simulink library "BLDC_controller_Lib"  (R2017b)
settings: Solver=VariableStepAuto  StartTime=0.0  StopTime=10.0  RelTol=1e-3
libraries: BLDC_controller_Lib x9, simulink x9
settings Model: Creator=37ef  LastModifiedBy=eferu

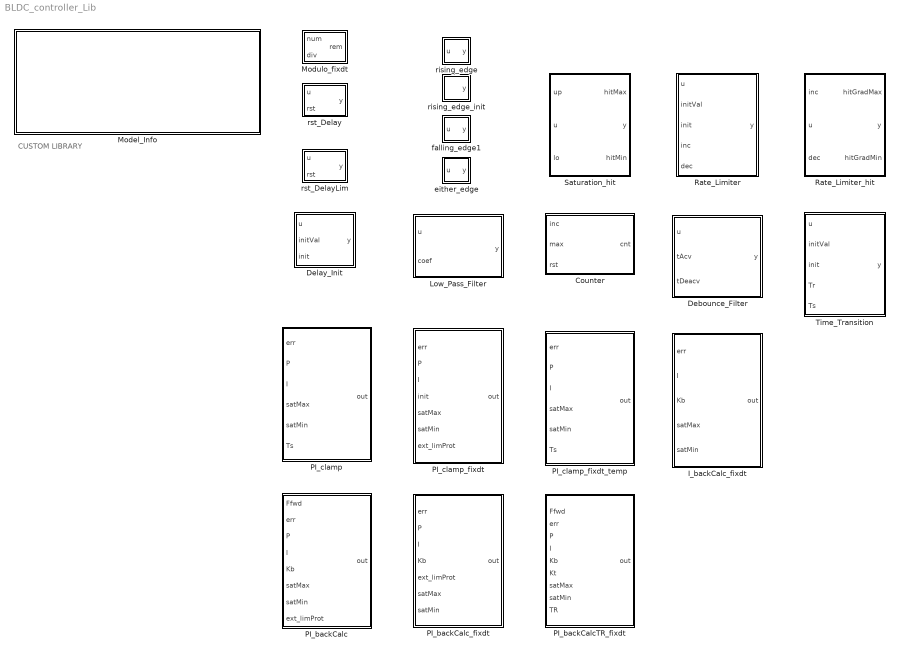
== system BLDC_controller_Lib ==
  note: CUSTOM LIBRARY
  Counter : Subsystem  TreatAsAtomicUnit=on  mask{z_cntInit=0}
      mask prompts: z_cntInit "Insert initial counter value"
      settings: AttributesFormatString=Ini=%<z_cntInit>  RTWFcnNameOpts=Use subsystem name
      mask Display: plot(0.15+[0.1,0.1],[0.1,0.9],[0.08,0.1,0.12]+0.15,[0.88,0.9,0.88],[0.25,0.8],[0.1,0.1],[0.88,0.9,0.88]-0.1,[0.08,0.1,0.12],0.05+[0.2,0.3,0.3,0.4,0.4,0.5,0.5,0.6,0.6,0.7],1.5*([0.1,0.1,0.2,0.2,0.3,0.3,0.4,0.4,0.5,0.5]-0.1)+0.1)
  Debounce_Filter : Subsystem  TreatAsAtomicUnit=on
      mask help:
      | This block implements a debounce filter.
      | The input and the output are boolean.
      | • Output will be 1 if input equals 1 during at least tAcv
      | • Output will be 0 if input equals 0 during at least tDeacv
      | ► Note that tAcv and tDeacv are integer numbers, represeting the number of time samples for Activation and Deactivation, respectively.
      settings: RTWFcnNameOpts=Use subsystem name
      mask Display:
      | plot([0.10 0.20 0.20 0.22 0.22 0.24 0.24 0.26 0.26 0.28 0.28 0.7 0.7 0.72 0.72 0.74 0.74 0.76 0.76 0.78 0.78 0.9],0.2+0.75*[0.55 0.55 0.9 0.9 0.55 0.55 0.9 0.9 0.55 0.55 0.9 0.9 0.55 0.55 0.9 0.9 0.55 0.55 0.9 0.9 0.55 0.55])
      | 
      | plot([0.10 0.28 0.28 0.78 0.78 0.90],0.2+0.7*[0.1 0.1 0.45 0.45 0.1 0.1])
  Delay_Init : Subsystem  mask{initVal=0}
      mask prompts: initVal "Initial value at program start"
      settings: AttributesFormatString=Ini=%<initVal>
      mask Display: dpoly(1,[1 0],'z')
  I_backCalc_fixdt : Subsystem  TreatAsAtomicUnit=on  mask{yInit=0}
      mask prompts: yInit "Initial output"
      settings: AttributesFormatString=Ini=%<yInit>  RTWFcnNameOpts=Use subsystem name
      mask Display: disp('I(z)')
  Low_Pass_Filter : Subsystem  TreatAsAtomicUnit=on
      settings: RTWFcnNameOpts=Use subsystem name
      mask Display:
      | plot(0,0,100,100, ...
      | [73,75,73,75,25,25,28,25,22,25],[18,20,22,20,20,84,82,84,82,84], ...
      | [25,33,33,72],[20,20,70,70],[33,34,36,39,44,50,56,66,73],[20,25,33,43,55,63,66,70,70]);
      | text(50,40,'coef'),
  Model_Info : Subsystem
      mask DialogControl DescGroupVar Prompt: Model info
      mask DialogControl DescTextVar Prompt: This mask gives quick information about the model.
      mask Display:
      | info = Simulink.MDLInfo(bdroot);
      | file = dir([bdroot '.slx']);
      | % image('logo.png', [0.48, 0.55, 0.5, 0.4]);
      | text(0.05, 0.5, [...
      |         'MODEL INFO \n\n' ...
      |         'Version: ' info.ModelVersion '\n' ...
      |         'Author: ' 'Emanuel Feru' '\n' ...
      |         'Last modified by: ' info.LastModifiedBy '\n' ...
      |         'Last update: ' file.date '\n\n'], ...
      |         'horizontalAlignment', 'left', ...
      |         'verticalAlignment', 'middle');
      | 
      | color('blue');
      | text(0.95, 0.08, [...
      |         'Copyright © 2019-2021 Emanuel FERU'], ...
      |         'horizontalAlignment', 'right', ...
      |         'verticalAlignment', 'bottom');
  Modulo_fixdt : Subsystem
  PI_backCalc : Subsystem  TreatAsAtomicUnit=on
      settings: RTWFcnNameOpts=Use subsystem name
      mask Display: disp('PI(z)')
  PI_backCalcTR_fixdt : Subsystem  TreatAsAtomicUnit=on
      settings: RTWFcnNameOpts=Use subsystem name
      mask Display: disp('PI(z)')
  PI_backCalc_fixdt : Subsystem  TreatAsAtomicUnit=on
      settings: RTWFcnNameOpts=Use subsystem name
      mask Display: disp('PI(z)')
  PI_clamp : Subsystem  TreatAsAtomicUnit=on
      settings: RTWFcnNameOpts=Use subsystem name
      mask Display: disp('PI(z)')
  PI_clamp_fixdt : Subsystem  TreatAsAtomicUnit=on
      settings: RTWFcnNameOpts=Use subsystem name
      mask Display: disp('PI(z)')
  PI_clamp_fixdt_temp : Subsystem  TreatAsAtomicUnit=on
      settings: RTWFcnNameOpts=Use subsystem name
      mask Display: disp('PI(z)')
  Rate_Limiter : Subsystem  TreatAsAtomicUnit=on
      settings: RTWFcnNameOpts=Use subsystem name
      mask Display: plot([0.15 0.85],[0.5 0.5],[0.5 0.5],[0.1 0.9],[0.25 0.75],[0.1 0.9])
  Rate_Limiter_hit : Subsystem  TreatAsAtomicUnit=on
      settings: RTWFcnNameOpts=Use subsystem name
      mask Display: plot([0.15 0.85],[0.5 0.5],[0.5 0.5],[0.1 0.9],[0.25 0.75],[0.1 0.9])
  Saturation_hit : Subsystem
      mask Display: plot([0.2 0.8],[0.5 0.5],[0.5 0.5],[0.05 0.95],[0.2 0.3 0.7 0.8],[0.05 0.05 0.95 0.95])
  Time_Transition : Subsystem  TreatAsAtomicUnit=on  mask{eps=5}
      mask prompts: eps "Convergence tolerance (eps)"
      mask help:
      | This block can be used to avoid discontinuity between a new input (discontinuous) and the previous output.
      |
      | When the input "init" is triggered, the error between "u" and "initVal" is set. This error is then reduced to 0 with respect to the transition time "Tr". When the error goes below a certain tolerance "eps", then the transition is finished.
      |
      | Once the error has been completely canceled (reduced to 0), then the output is equal to the input (without any slope constraint).
      settings: AttributesFormatString=eps=%<eps>  RTWFcnNameOpts=Use subsystem name
      mask Display:
      | plot(0,0,100,100,[88,90,88,90,29,29,31,29,27,29],[19,20,21,20,20,84,82,84,82,84]-5,...
      |     [35,40,50,60,70,85],[50,51,54,60,70,85]-5,[35,40,50,60,70,85],[30,35,45,56,70,85]-5);
      | text(35,22,'← Tr →');
  either_edge : Subsystem  StopFcn=%tagged  TreatAsAtomicUnit=on  mask(Either edge detection){}
      mask help:
      | Rising or falling edge detection for a logic signal.
      | When a rising or a falling edge on the input signal is detected, the output switches to 1 during one time step.
      mask Display: plot(0,0,100,100, [50 75 75 90], [90 90 10 10], [65 75 85], [55 45 55], [10 25 25 50], [10 10 90 90], [15 25 35], [45 55 45] )
  falling_edge1 : Subsystem  StopFcn=%tagged  TreatAsAtomicUnit=on  mask(Falling edge detection){}
      mask help:
      | Falling edge detection for a logic signal.
      | When a falling edge on the input signal is detected, the output switches to 1 during one time step.
      mask Display: plot(0,0,100,100, [20 50 50 80], [90 90 10 10], [40 50 60], [55 45 55] )
  rising_edge : Subsystem  StopFcn=%tagged  TreatAsAtomicUnit=on  mask(Rising edge detection){}
      mask help:
      | Rising edge detection for a logic signal.
      | When a rising edge on the input signal is detected, the output switches to 1 during one time step.
      mask Display: plot(0,0,100,100, [20 50 50 80], [10 10 90 90], [40 50 60], [45 55 45] )
  rising_edge_init : Subsystem  StopFcn=%tagged  TreatAsAtomicUnit=on  mask(Rising edge init){}
      mask help:
      | Rising edge at init of the subsystem.
      | This block can be used for example in action subsystem to create a trig when function is called.
      mask Display: plot(0,0,100,100, [20 50 50 80], [10 10 90 90], [40 50 60], [45 55 45] )
  rst_Delay : Subsystem  mask{initVal=0}
      mask prompts: initVal "Initial value at program start"
      settings: AttributesFormatString=Ini=%<InitVal>
      mask Display: dpoly(1,[1 0],'z')
  rst_DelayLim : Subsystem  mask{z_cntMaxLim=200}
      mask prompts: z_cntMaxLim "Maximum counter limit"
      settings: AttributesFormatString=Ini=%<z_cntMaxLim>
      mask Display: dpoly(1,[1 0],'z')

== system BLDC_controller_Lib/Counter ==
  inc : Inport
  max : Inport  Port=2
  rst : Inport  Port=3
  MinMax : MinMax  Inputs=2
  Sum1 : Sum  Inputs=|++  RndMeth=Simplest  InputSameDT=on  OutDataTypeStr=Inherit: Same as first input
  rst_Delay : BLDC_controller_Lib/rst_Delay  initVal=z_cntInit
      settings: AttributesFormatString=Ini=%<InitVal>
  cnt : Outport
  wires:
  inc/1 -> Sum1/1
  rst/1 -> rst_Delay/2
  Sum1/1 -> cnt/1, MinMax/1
  max/1 -> MinMax/2
  MinMax/1 -> rst_Delay/1
  rst_Delay/1 -> Sum1/2

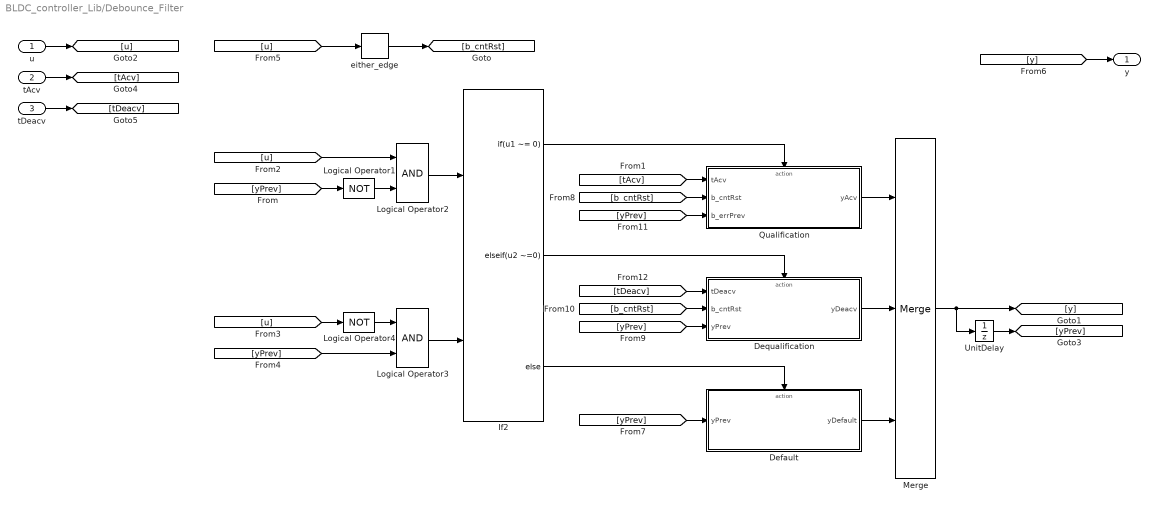
== system BLDC_controller_Lib/Debounce_Filter ==
  u : Inport
  tAcv : Inport  Port=2
  tDeacv : Inport  Port=3
  Default : Subsystem
  Dequalification : Subsystem
  If2 : If  NumInputs=2  IfExpression=u1 ~= 0  ElseIfExpressions=u2 ~=0
  Logical Operator1 : Logic  Operator=NOT  AllPortsSameDT=off  OutDataTypeStr=boolean
  Logical Operator2 : Logic  AllPortsSameDT=off  OutDataTypeStr=boolean
  Logical Operator3 : Logic  AllPortsSameDT=off  OutDataTypeStr=boolean
  Logical Operator4 : Logic  Operator=NOT  AllPortsSameDT=off  OutDataTypeStr=boolean
  Merge : Merge  Inputs=3
  Qualification : Subsystem
  UnitDelay : UnitDelay  SampleTime=-1
      settings: AttributesFormatString=Ini=%<X0>
  either_edge : BLDC_controller_Lib/either_edge
  y : Outport
  wires:
  Logical Operator2/1 -> If2/1
  Logical Operator3/1 -> If2/2
  [b_cntRst] -> Dequalification/2(b_cntRst)
  [yPrev] -> Logical Operator3/2
  Logical Operator4/1 -> Logical Operator3/1
  [tDeacv] -> Dequalification/1(tDeacv)
  Merge/1 -> UnitDelay/1, [y]
  UnitDelay/1 -> [yPrev]
  [b_cntRst] -> Qualification/2(b_cntRst)
  [tAcv] -> Qualification/1(tAcv)
  Dequalification/1(yDeacv) -> Merge/2
  Default/1(yDefault) -> Merge/3
  [yPrev] -> Qualification/3(b_errPrev)
  If2/2 -> Dequalification/Action
  [yPrev] -> Default/1(yPrev)
  [u] -> either_edge/1
  [y] -> y/1
  u/1 -> [u]
  If2/3 -> Default/Action
  [yPrev] -> Dequalification/3(yPrev)
  [u] -> Logical Operator4/1
  [yPrev] -> Logical Operator1/1
  Logical Operator1/1 -> Logical Operator2/2
  [u] -> Logical Operator2/1
  Qualification/1(yAcv) -> Merge/1
  If2/1 -> Qualification/Action
  tAcv/1 -> [tAcv]
  tDeacv/1 -> [tDeacv]
  either_edge/1 -> [b_cntRst]

== system BLDC_controller_Lib/Delay_Init ==
  u : Inport
  initVal : Inport  Port=2
  init : Inport  Port=3
  Switch1 : Switch  Criteria=u2 ~= 0  OutDataTypeStr=Inherit: Inherit via back propagation  RndMeth=Simplest  InputSameDT=on
  Switch2 : Switch  Criteria=u2 ~= 0  OutDataTypeStr=Inherit: Inherit via back propagation  RndMeth=Simplest  InputSameDT=on
  UnitDelay : UnitDelay  InitialCondition=initVal  SampleTime=-1
      settings: AttributesFormatString=Ini=%<X0>
  y : Outport
  wires:
  UnitDelay/1 -> Switch1/3
  Switch1/1 -> y/1
  init/1 -> Switch1/2, Switch2/2
  Switch2/1 -> UnitDelay/1
  u/1 -> Switch2/3
  initVal/1 -> Switch2/1, Switch1/1

== system BLDC_controller_Lib/I_backCalc_fixdt ==
  err : Inport
  I : Inport  Port=2
  Kb : Inport  Port=3
  satMax : Inport  Port=4
  satMin : Inport  Port=5
  Divide1 : Product  Inputs=**  RndMeth=Simplest
  Divide2 : Product  Inputs=**  RndMeth=Simplest
  Integrator : Subsystem
  Saturation Dynamic1 : simulink/Discontinuities/Saturation Dynamic  OutMin=[]  OutMax=[]  OutDataTypeStr=Inherit: Same as second input  OutDataType=fixdt(1, 16)  OutScaling=2^-10  DoSatur=off
  Sum2 : Sum  RndMeth=Simplest  SaturateOnIntegerOverflow=on
  Sum3 : Sum  Inputs=-+|  RndMeth=Simplest
  UnitDelay : UnitDelay  SampleTime=-1
      settings: AttributesFormatString=Ini=%<X0>
  out : Outport
  wires:
  satMin/1 -> Saturation Dynamic1/3
  satMax/1 -> Saturation Dynamic1/1
  I/1 -> Divide2/2
  err/1 -> Divide2/1
  Saturation Dynamic1/1 -> Sum3/2, out/1
  Integrator/1(y) -> Sum3/1, Saturation Dynamic1/2
  UnitDelay/1 -> Sum2/2
  Divide1/1 -> UnitDelay/1
  Sum3/1 -> Divide1/1
  Kb/1 -> Divide1/2
  Divide2/1 -> Sum2/1
  Sum2/1 -> Integrator/1(u)

== system BLDC_controller_Lib/Low_Pass_Filter ==
  u : Inport
  coef : Inport  Port=2
  Data Type Conversion : DataTypeConversion  OutDataTypeStr=fixdt(1,16,4)
  Divide3 : Product  Inputs=**  RndMeth=Simplest
  Sum2 : Sum  Inputs=+-  RndMeth=Simplest  SaturateOnIntegerOverflow=on  OutDataTypeStr=Inherit: Same as first input
  Sum3 : Sum  RndMeth=Simplest  OutDataTypeStr=Inherit: Same as first input
  UnitDelay1 : UnitDelay  SampleTime=-1
  y : Outport
  wires:
  Sum3/1 -> Data Type Conversion/1, UnitDelay1/1
  Sum2/1 -> Divide3/2
  UnitDelay1/1 -> Sum3/2, Sum2/2
  Data Type Conversion/1 -> y/1
  u/1 -> Sum2/1
  Divide3/1 -> Sum3/1
  coef/1 -> Divide3/1

== system BLDC_controller_Lib/Model_Info ==

== system BLDC_controller_Lib/Modulo_fixdt ==
  note: Modulo implementation: rem = num - div*(num/div)
      | Note : Division and multiplier has the setting 'Floor'
  num : Inport
  div : Inport  Port=2
  Divide2 : Product  Inputs=*/  OutDataTypeStr=fixdt(1,16,0)
  Divide3 : Product  Inputs=**  OutDataTypeStr=Inherit: Same as first input
  Sum3 : Sum  Inputs=|+-  RndMeth=Simplest  OutDataTypeStr=Inherit: Same as first input
  rem : Outport
  wires:
  Divide3/1 -> Sum3/2
  num/1 -> Divide2/1, Sum3/1
  Sum3/1 -> rem/1
  div/1 -> Divide2/2, Divide3/2
  Divide2/1 -> Divide3/1

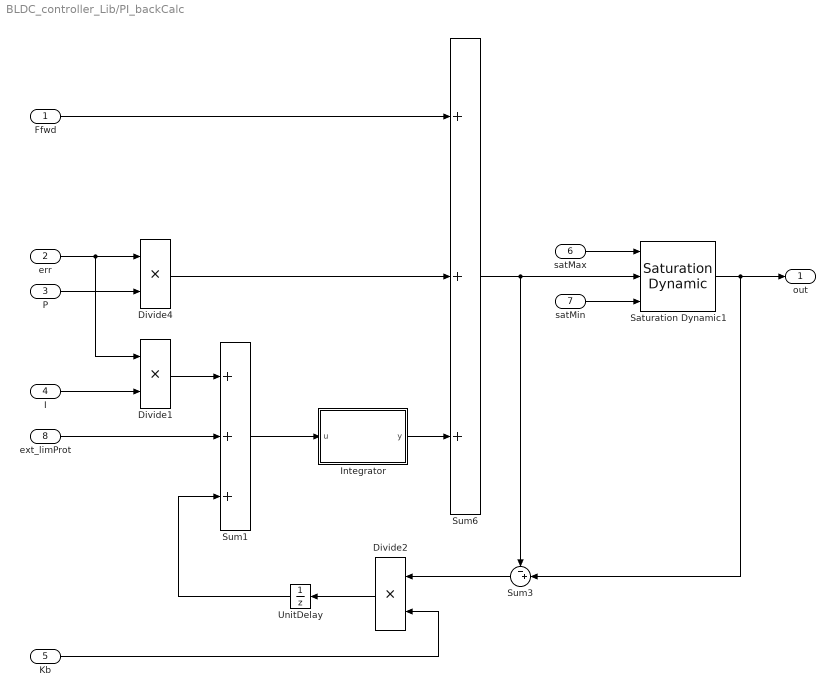
== system BLDC_controller_Lib/PI_backCalc ==
  Ffwd : Inport
  err : Inport  Port=2
  P : Inport  Port=3
  I : Inport  Port=4
  Kb : Inport  Port=5
  satMax : Inport  Port=6
  satMin : Inport  Port=7
  ext_limProt : Inport  Port=8
  Divide1 : Product  Inputs=**  RndMeth=Simplest
  Divide2 : Product  Inputs=**  RndMeth=Simplest
  Divide4 : Product  Inputs=**  RndMeth=Simplest
  Integrator : Subsystem
  Saturation Dynamic1 : simulink/Discontinuities/Saturation Dynamic  OutMin=[]  OutMax=[]  OutDataTypeStr=Inherit: Same as second input  OutDataType=fixdt(1, 16)  OutScaling=2^-10  DoSatur=off
  Sum1 : Sum  Inputs=+++  OutDataTypeStr=Inherit: Inherit via back propagation  RndMeth=Simplest  SaturateOnIntegerOverflow=on
  Sum3 : Sum  Inputs=-+|  OutDataTypeStr=Inherit: Inherit via back propagation  RndMeth=Simplest  SaturateOnIntegerOverflow=on
  Sum6 : Sum  Inputs=+++  OutDataTypeStr=single  RndMeth=Simplest  SaturateOnIntegerOverflow=on
  UnitDelay : UnitDelay  SampleTime=-1
      settings: AttributesFormatString=Ini=%<X0>
  out : Outport
  wires:
  I/1 -> Divide1/2
  P/1 -> Divide4/2
  Integrator/1(y) -> Sum6/3
  Saturation Dynamic1/1 -> Sum3/2, out/1
  Sum1/1 -> Integrator/1(u)
  Divide4/1 -> Sum6/2
  err/1 -> Divide1/1, Divide4/1
  satMax/1 -> Saturation Dynamic1/1
  Sum6/1 -> Sum3/1, Saturation Dynamic1/2
  satMin/1 -> Saturation Dynamic1/3
  Divide1/1 -> Sum1/1
  UnitDelay/1 -> Sum1/3
  Divide2/1 -> UnitDelay/1
  Sum3/1 -> Divide2/1
  Kb/1 -> Divide2/2
  ext_limProt/1 -> Sum1/2
  Ffwd/1 -> Sum6/1

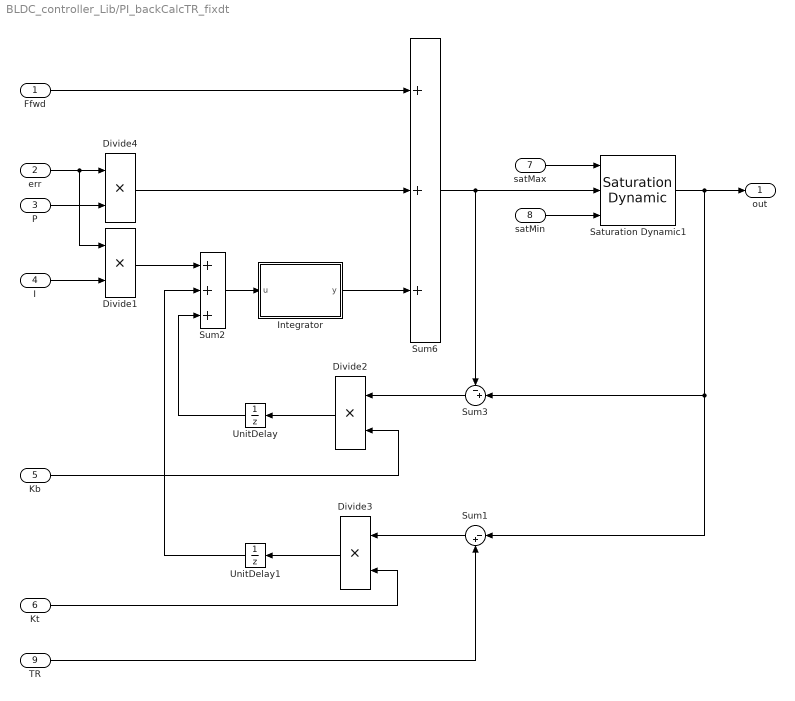
== system BLDC_controller_Lib/PI_backCalcTR_fixdt ==
  Ffwd : Inport
  err : Inport  Port=2
  P : Inport  Port=3
  I : Inport  Port=4
  Kb : Inport  Port=5
  Kt : Inport  Port=6
  satMax : Inport  Port=7
  satMin : Inport  Port=8
  TR : Inport  Port=9
  Divide{1..4} (4 alike) : Product  Inputs=**  RndMeth=Simplest
  Integrator : Subsystem
  Saturation Dynamic1 : simulink/Discontinuities/Saturation Dynamic  OutMin=[]  OutMax=[]  OutDataTypeStr=Inherit: Same as second input  OutDataType=fixdt(1, 16)  OutScaling=2^-10  DoSatur=off
  Sum1 : Sum  Inputs=|-+  RndMeth=Simplest  SaturateOnIntegerOverflow=on
  Sum2 : Sum  Inputs=+++  RndMeth=Simplest  SaturateOnIntegerOverflow=on
  Sum3 : Sum  Inputs=-+|  RndMeth=Simplest  SaturateOnIntegerOverflow=on
  Sum6 : Sum  Inputs=+++  OutDataTypeStr=fixdt(1,16,4)  RndMeth=Simplest  SaturateOnIntegerOverflow=on
  UnitDelay : UnitDelay  SampleTime=-1
      settings: AttributesFormatString=Ini=%<X0>
  UnitDelay1 : UnitDelay  SampleTime=-1
      settings: AttributesFormatString=Ini=%<X0>
  out : Outport
  wires:
  Sum2/1 -> Integrator/1(u)
  Kb/1 -> Divide2/2
  Saturation Dynamic1/1 -> out/1, Sum3/2, Sum1/1
  Sum6/1 -> Sum3/1, Saturation Dynamic1/2
  UnitDelay/1 -> Sum2/3
  Sum3/1 -> Divide2/1
  Divide2/1 -> UnitDelay/1
  Divide1/1 -> Sum2/1
  I/1 -> Divide1/2
  err/1 -> Divide1/1, Divide4/1
  Integrator/1(y) -> Sum6/3
  satMax/1 -> Saturation Dynamic1/1
  Divide4/1 -> Sum6/2
  satMin/1 -> Saturation Dynamic1/3
  P/1 -> Divide4/2
  Kt/1 -> Divide3/2
  Divide3/1 -> UnitDelay1/1
  Sum1/1 -> Divide3/1
  TR/1 -> Sum1/2
  UnitDelay1/1 -> Sum2/2
  Ffwd/1 -> Sum6/1

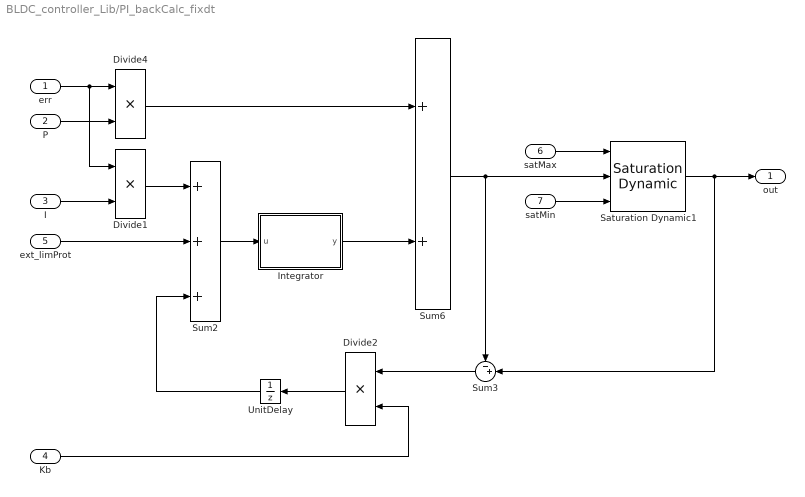
== system BLDC_controller_Lib/PI_backCalc_fixdt ==
  err : Inport
  P : Inport  Port=2
  I : Inport  Port=3
  Kb : Inport  Port=4
  ext_limProt : Inport  Port=5
  satMax : Inport  Port=6
  satMin : Inport  Port=7
  Divide1 : Product  Inputs=**  RndMeth=Simplest  SaturateOnIntegerOverflow=on
  Divide2 : Product  Inputs=**  RndMeth=Simplest
  Divide4 : Product  Inputs=**  OutDataTypeStr=fixdt(1,16,5)  RndMeth=Simplest  SaturateOnIntegerOverflow=on
  Integrator : Subsystem
  Saturation Dynamic1 : simulink/Discontinuities/Saturation Dynamic  OutMin=[]  OutMax=[]  OutDataTypeStr=Inherit: Same as second input  OutDataType=fixdt(1, 16)  OutScaling=2^-10  DoSatur=off
  Sum2 : Sum  Inputs=+++  RndMeth=Simplest  SaturateOnIntegerOverflow=on
  Sum3 : Sum  Inputs=-+|  RndMeth=Simplest
  Sum6 : Sum  OutDataTypeStr=fixdt(1,16,4)  RndMeth=Simplest  SaturateOnIntegerOverflow=on
  UnitDelay : UnitDelay  SampleTime=-1
      settings: AttributesFormatString=Ini=%<X0>
  out : Outport
  wires:
  ext_limProt/1 -> Sum2/2
  P/1 -> Divide4/2
  satMin/1 -> Saturation Dynamic1/3
  satMax/1 -> Saturation Dynamic1/1
  err/1 -> Divide4/1, Divide1/1
  I/1 -> Divide1/2
  Divide1/1 -> Sum2/1
  Divide2/1 -> UnitDelay/1
  Sum3/1 -> Divide2/1
  UnitDelay/1 -> Sum2/3
  Sum6/1 -> Saturation Dynamic1/2, Sum3/1
  Saturation Dynamic1/1 -> Sum3/2, out/1
  Kb/1 -> Divide2/2
  Sum2/1 -> Integrator/1(u)
  Integrator/1(y) -> Sum6/2
  Divide4/1 -> Sum6/1

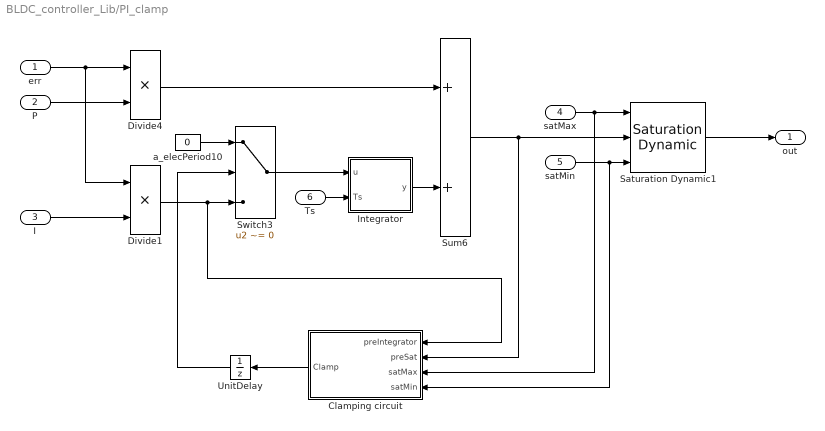
== system BLDC_controller_Lib/PI_clamp ==
  err : Inport
  P : Inport  Port=2
  I : Inport  Port=3
  satMax : Inport  Port=4
  satMin : Inport  Port=5
  Ts : Inport  Port=6
  Clamping circuit : Subsystem
  Divide1 : Product  Inputs=**  RndMeth=Simplest
  Divide4 : Product  Inputs=**  RndMeth=Simplest
  Integrator : Subsystem
  Saturation Dynamic1 : simulink/Discontinuities/Saturation Dynamic  OutMin=[]  OutMax=[]  OutDataTypeStr=Inherit: Same as second input  OutDataType=fixdt(1, 16)  OutScaling=2^-10  DoSatur=off
  Sum6 : Sum  OutDataTypeStr=single  RndMeth=Simplest  SaturateOnIntegerOverflow=on
  Switch3 : Switch  Criteria=u2 ~= 0  OutDataTypeStr=Inherit: Inherit via back propagation  RndMeth=Zero
  UnitDelay : UnitDelay  SampleTime=-1
      settings: AttributesFormatString=Ini=%<X0>
  a_elecPeriod10 : Constant  Value=0  OutDataTypeStr=Inherit: Inherit via back propagation
  out : Outport
  wires:
  satMin/1 -> Saturation Dynamic1/3, Clamping circuit/4(satMin)
  Sum6/1 -> Saturation Dynamic1/2, Clamping circuit/2(preSat)
  satMax/1 -> Saturation Dynamic1/1, Clamping circuit/3(satMax)
  Divide1/1 -> Switch3/3, Clamping circuit/1(preIntegrator)
  UnitDelay/1 -> Switch3/2
  Clamping circuit/1(Clamp) -> UnitDelay/1
  err/1 -> Divide4/1, Divide1/1
  Divide4/1 -> Sum6/1
  a_elecPeriod10/1 -> Switch3/1
  Switch3/1 -> Integrator/1(u)
  Saturation Dynamic1/1 -> out/1
  Integrator/1(y) -> Sum6/2
  P/1 -> Divide4/2
  I/1 -> Divide1/2
  Ts/1 -> Integrator/2(Ts)

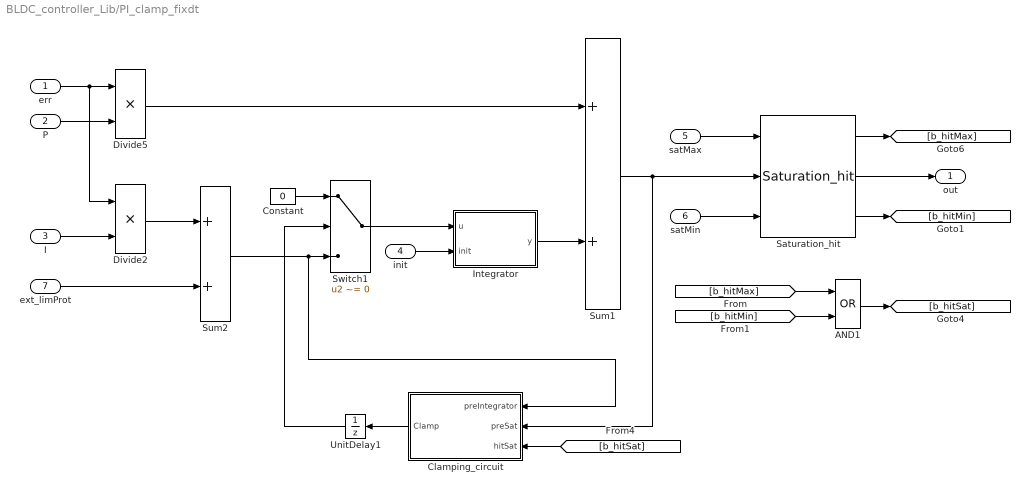
== system BLDC_controller_Lib/PI_clamp_fixdt ==
  err : Inport
  P : Inport  Port=2
  I : Inport  Port=3
  init : Inport  Port=4
  satMax : Inport  Port=5
  satMin : Inport  Port=6
  ext_limProt : Inport  Port=7
  AND1 : Logic  DisableCoverage=on  Operator=OR  OutDataTypeStr=boolean
  Clamping_circuit : Subsystem
  Constant : Constant  Value=0  OutDataTypeStr=Inherit: Inherit via back propagation
  Divide2 : Product  Inputs=**  RndMeth=Simplest
  Divide5 : Product  Inputs=**  OutDataTypeStr=fixdt(1,16,5)  RndMeth=Simplest  SaturateOnIntegerOverflow=on
  Integrator : Subsystem
  Saturation_hit : BLDC_controller_Lib/Saturation_hit  SystemSampleTime=-1
  Sum1 : Sum  OutDataTypeStr=fixdt(1,16,4)  RndMeth=Simplest  SaturateOnIntegerOverflow=on
  Sum2 : Sum  RndMeth=Simplest  SaturateOnIntegerOverflow=on
  Switch1 : Switch  Criteria=u2 ~= 0  OutDataTypeStr=Inherit: Inherit via back propagation  RndMeth=Zero
  UnitDelay1 : UnitDelay  SampleTime=-1
      settings: AttributesFormatString=Ini=%<X0>
  out : Outport
  wires:
  err/1 -> Divide5/1, Divide2/1
  ext_limProt/1 -> Sum2/2
  Divide2/1 -> Sum2/1
  Divide5/1 -> Sum1/1
  I/1 -> Divide2/2
  Integrator/1(y) -> Sum1/2
  P/1 -> Divide5/2
  satMax/1 -> Saturation_hit/1
  satMin/1 -> Saturation_hit/3
  Saturation_hit/1 -> [b_hitMax]
  Saturation_hit/3 -> [b_hitMin]
  Constant/1 -> Switch1/1
  Sum1/1 -> Clamping_circuit/2(preSat), Saturation_hit/2
  Sum2/1 -> Clamping_circuit/1(preIntegrator), Switch1/3
  Switch1/1 -> Integrator/1(u)
  Clamping_circuit/1(Clamp) -> UnitDelay1/1
  UnitDelay1/1 -> Switch1/2
  [b_hitMax] -> AND1/1
  [b_hitMin] -> AND1/2
  AND1/1 -> [b_hitSat]
  [b_hitSat] -> Clamping_circuit/3(hitSat)
  Saturation_hit/2 -> out/1
  init/1 -> Integrator/2(init)

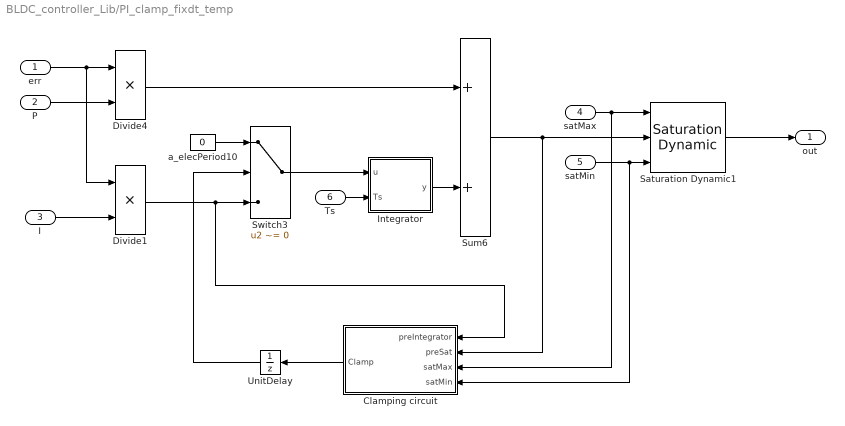
== system BLDC_controller_Lib/PI_clamp_fixdt_temp ==
  err : Inport
  P : Inport  Port=2
  I : Inport  Port=3
  satMax : Inport  Port=4
  satMin : Inport  Port=5
  Ts : Inport  Port=6
  Clamping circuit : Subsystem
  Divide1 : Product  Inputs=**  RndMeth=Simplest
  Divide4 : Product  Inputs=**  RndMeth=Simplest
  Integrator : Subsystem
  Saturation Dynamic1 : simulink/Discontinuities/Saturation Dynamic  OutMin=[]  OutMax=[]  OutDataTypeStr=Inherit: Same as second input  OutDataType=fixdt(1, 16)  OutScaling=2^-10  DoSatur=off
  Sum6 : Sum  OutDataTypeStr=fixdt(1,16,4)  RndMeth=Simplest  SaturateOnIntegerOverflow=on
  Switch3 : Switch  Criteria=u2 ~= 0  OutDataTypeStr=Inherit: Inherit via back propagation  RndMeth=Zero
  UnitDelay : UnitDelay  SampleTime=-1
      settings: AttributesFormatString=Ini=%<X0>
  a_elecPeriod10 : Constant  Value=0  OutDataTypeStr=Inherit: Inherit via back propagation
  out : Outport
  wires:
  UnitDelay/1 -> Switch3/2
  Clamping circuit/1(Clamp) -> UnitDelay/1
  Divide1/1 -> Switch3/3, Clamping circuit/1(preIntegrator)
  Switch3/1 -> Integrator/1(u)
  I/1 -> Divide1/2
  err/1 -> Divide4/1, Divide1/1
  Integrator/1(y) -> Sum6/2
  Sum6/1 -> Clamping circuit/2(preSat), Saturation Dynamic1/2
  satMax/1 -> Saturation Dynamic1/1, Clamping circuit/3(satMax)
  Divide4/1 -> Sum6/1
  satMin/1 -> Saturation Dynamic1/3, Clamping circuit/4(satMin)
  a_elecPeriod10/1 -> Switch3/1
  Saturation Dynamic1/1 -> out/1
  P/1 -> Divide4/2
  Ts/1 -> Integrator/2(Ts)

== system BLDC_controller_Lib/Rate_Limiter ==
  note: Rate Limiter
      | Note: The sample time must be included in the Increment and Decrement values.
  u : Inport
  initVal : Inport  Port=2
  init : Inport  Port=3
  inc : Inport  Port=4
  dec : Inport  Port=5
  Delay_Init1 : BLDC_controller_Lib/Delay_Init  initVal=0
  Saturation Dynamic : simulink/Discontinuities/Saturation Dynamic  OutMin=[]  OutMax=[]  OutDataTypeStr=Inherit: Same as second input  OutDataType=fixdt(1, 16)  OutScaling=2^-10  DoSatur=off
  Sum1 : Sum  Inputs=+-  RndMeth=Zero  OutDataTypeStr=Inherit: Same as first input
  Sum2 : Sum  RndMeth=Zero  OutDataTypeStr=Inherit: Same as first input
  y : Outport
  wires:
  Saturation Dynamic/1 -> Sum2/1
  initVal/1 -> Delay_Init1/2
  dec/1 -> Saturation Dynamic/3
  Sum1/1 -> Saturation Dynamic/2
  Sum2/1 -> y/1, Delay_Init1/1
  inc/1 -> Saturation Dynamic/1
  u/1 -> Sum1/1
  Delay_Init1/1 -> Sum2/2, Sum1/2
  init/1 -> Delay_Init1/3

== system BLDC_controller_Lib/Rate_Limiter_hit ==
  note: Rate Limiter
      | Note: The sample time must be included in the Increment and Decrement values.
  inc : Inport
  u : Inport  Port=2
  dec : Inport  Port=3
  Saturation_hit : BLDC_controller_Lib/Saturation_hit  SystemSampleTime=-1
  Sum1 : Sum  Inputs=+-  RndMeth=Zero  OutDataTypeStr=Inherit: Same as first input
  Sum2 : Sum  RndMeth=Zero  OutDataTypeStr=Inherit: Same as first input
  UnitDelay : UnitDelay  SampleTime=-1
      settings: AttributesFormatString=Ini=%<X0>
  hitGradMax : Outport
  y : Outport  Port=2
  hitGradMin : Outport  Port=3
  wires:
  UnitDelay/1 -> Sum1/2, Sum2/2
  u/1 -> Sum1/1
  inc/1 -> Saturation_hit/1
  Sum2/1 -> UnitDelay/1, y/1
  Sum1/1 -> Saturation_hit/2
  dec/1 -> Saturation_hit/3
  Saturation_hit/2 -> Sum2/1
  Saturation_hit/1 -> hitGradMax/1
  Saturation_hit/3 -> hitGradMin/1

== system BLDC_controller_Lib/Saturation_hit ==
  up : Inport
  u : Inport  Port=2
  lo : Inport  Port=3
  LowerRelop1 : RelationalOperator  DisableCoverage=on  Operator=>  OutDataTypeStr=boolean  RndMeth=Nearest
  Switch1 : Switch  Criteria=u2 ~= 0  OutDataTypeStr=Inherit: Inherit via back propagation  RndMeth=Zero
  Switch3 : Switch  Criteria=u2 ~= 0  OutDataTypeStr=Inherit: Inherit via back propagation  RndMeth=Zero
  UpperRelop : RelationalOperator  DisableCoverage=on  Operator=<  OutDataTypeStr=boolean  RndMeth=Nearest
  hitMax : Outport
  y : Outport  Port=2
  hitMin : Outport  Port=3
  wires:
  Switch1/1 -> y/1
  u/1 -> Switch3/3, LowerRelop1/1, UpperRelop/1
  up/1 -> LowerRelop1/2, Switch1/1
  UpperRelop/1 -> Switch3/2, hitMin/1
  LowerRelop1/1 -> hitMax/1, Switch1/2
  lo/1 -> Switch3/1, UpperRelop/2
  Switch3/1 -> Switch1/3

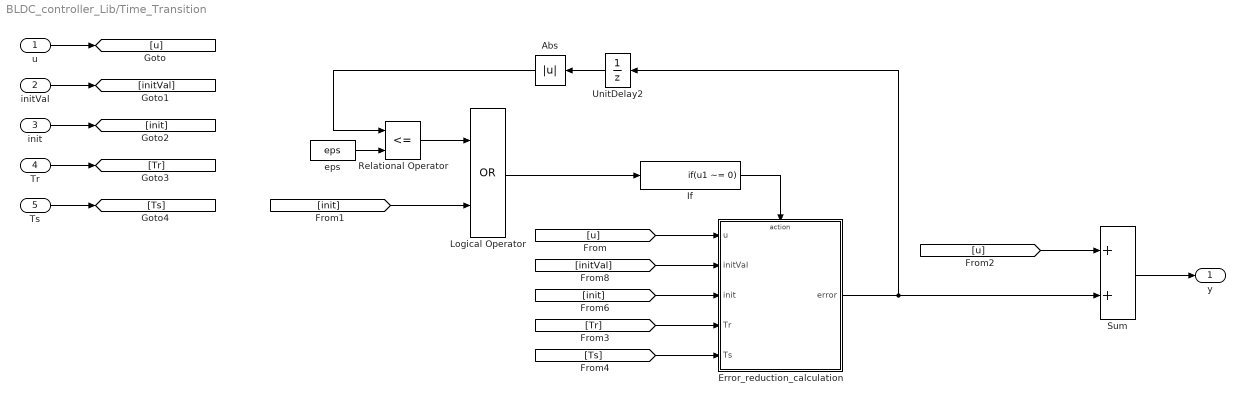
== system BLDC_controller_Lib/Time_Transition ==
  u : Inport
  initVal : Inport  Port=2
  init : Inport  Port=3
  Tr : Inport  Port=4
  Ts : Inport  Port=5
  Abs : Abs  RndMeth=Zero  SaturateOnIntegerOverflow=on
  Error_reduction_calculation : Subsystem  TreatAsAtomicUnit=on
  If : If  IfExpression=u1 ~= 0  ShowElse=off
  Logical Operator : Logic  Operator=OR  OutDataTypeStr=boolean
  Relational Operator : RelationalOperator  Operator=<=  OutDataTypeStr=boolean  RndMeth=Nearest  InputSameDT=on
  Sum : Sum  RndMeth=Zero  SaturateOnIntegerOverflow=on  OutDataTypeStr=Inherit: Same as first input
  UnitDelay2 : UnitDelay  SampleTime=-1
      settings: AttributesFormatString=Ini=%<X0>
  eps : Constant  Value=eps  OutDataTypeStr=Inherit: Inherit via back propagation
  y : Outport
  wires:
  eps/1 -> Relational Operator/2
  Error_reduction_calculation/1(error) -> Sum/2, UnitDelay2/1
  UnitDelay2/1 -> Abs/1
  Logical Operator/1 -> If/1
  [init] -> Logical Operator/2
  Relational Operator/1 -> Logical Operator/1
  If/1 -> Error_reduction_calculation/Action
  Abs/1 -> Relational Operator/1
  Sum/1 -> y/1
  u/1 -> [u]
  [u] -> Error_reduction_calculation/1(u)
  initVal/1 -> [initVal]
  [initVal] -> Error_reduction_calculation/2(initVal)
  [init] -> Error_reduction_calculation/3(init)
  init/1 -> [init]
  [Tr] -> Error_reduction_calculation/4(Tr)
  Tr/1 -> [Tr]
  Ts/1 -> [Ts]
  [Ts] -> Error_reduction_calculation/5(Ts)
  [u] -> Sum/1

== system BLDC_controller_Lib/either_edge ==
  u : Inport
  Relational Operator : RelationalOperator  Operator=~=  OutDataTypeStr=boolean  RndMeth=Nearest  InputSameDT=on
  UnitDelay : UnitDelay  SampleTime=-1
      settings: AttributesFormatString=Ini=%<X0>
  y : Outport
  wires:
  UnitDelay/1 -> Relational Operator/2
  Relational Operator/1 -> y/1
  u/1 -> UnitDelay/1, Relational Operator/1

== system BLDC_controller_Lib/falling_edge1 ==
  u : Inport
  Logical Operator : Logic  Tag=struct('inputs','2','comment',struct('text','','placement',1),'logdata',struct('maxnumvals',inf,'plotchannels',[],'loggingmode',3,'channels',1),'operator','AND','output',struct('variable','','description','','name','$S_$B','address','','class','default','type','Bool','unit',''),'scalingvalid',0,'date',733067.68453166669)  OutDataTypeStr=boolean
  Logical Operator1 : Logic  Tag=struct('inputs','1','comment',struct('text','','placement',1),'logdata',struct('maxnumvals',inf,'plotchannels',[],'loggingmode',3,'channels',1),'operator','NOT','output',struct('variable','','description','','name','$S_$B','address','','class','default','type','Bool','unit',''),'scalingvalid',0,'date',733067.68453201384)  Operator=NOT  Inputs=1  OutDataTypeStr=boolean
  UnitDelay : UnitDelay  SampleTime=-1
      settings: AttributesFormatString=Ini=%<X0>
  y : Outport
  wires:
  UnitDelay/1 -> Logical Operator/2
  Logical Operator1/1 -> Logical Operator/1
  u/1 -> UnitDelay/1, Logical Operator1/1
  Logical Operator/1 -> y/1

== system BLDC_controller_Lib/rising_edge ==
  u : Inport
  Logical Operator : Logic  Tag=struct('inputs','2','comment',struct('text','','placement',1),'logdata',struct('maxnumvals',inf,'plotchannels',[],'loggingmode',3,'channels',1),'operator','AND','output',struct('variable','','description','','name','$S_$B','address','','class','default','type','Bool','unit',''),'scalingvalid',0,'date',733067.68458487268)  OutDataTypeStr=boolean
  Logical Operator1 : Logic  Tag=struct('inputs','1','comment',struct('text','','placement',1),'logdata',struct('maxnumvals',inf,'plotchannels',[],'loggingmode',3,'channels',1),'operator','NOT','output',struct('variable','','description','','name','$S_$B','address','','class','default','type','Bool','unit',''),'scalingvalid',0,'date',733067.68458533566)  Operator=NOT  Inputs=1  OutDataTypeStr=boolean
  UnitDelay : UnitDelay  SampleTime=-1
      settings: AttributesFormatString=Ini=%<X0>
  y : Outport
  wires:
  UnitDelay/1 -> Logical Operator1/1
  Logical Operator1/1 -> Logical Operator/2
  u/1 -> Logical Operator/1, UnitDelay/1
  Logical Operator/1 -> y/1

== system BLDC_controller_Lib/rising_edge_init ==
  Constant : Constant  Value=0  OutDataTypeStr=boolean
  UnitDelay : UnitDelay  InitialCondition=1  SampleTime=-1
      settings: AttributesFormatString=Ini=%<X0>
  y : Outport
  wires:
  Constant/1 -> UnitDelay/1
  UnitDelay/1 -> y/1

== system BLDC_controller_Lib/rst_Delay ==
  u : Inport
  rst : Inport  Port=2
  Constant23 : Constant  Value=0  OutDataTypeStr=Inherit: Inherit via back propagation
  Switch1 : Switch  Criteria=u2 ~= 0  OutDataTypeStr=Inherit: Inherit via back propagation  RndMeth=Simplest
  UnitDelay : UnitDelay  InitialCondition=initVal  SampleTime=-1
      settings: AttributesFormatString=Ini=%<X0>
  y : Outport
  wires:
  Switch1/1 -> y/1
  u/1 -> UnitDelay/1
  UnitDelay/1 -> Switch1/3
  rst/1 -> Switch1/2
  Constant23/1 -> Switch1/1

== system BLDC_controller_Lib/rst_DelayLim ==
  u : Inport
  rst : Inport  Port=2
  Constant1 : Constant  Value=z_cntMaxLim  OutDataTypeStr=Inherit: Inherit via back propagation
  Constant23 : Constant  Value=0  OutDataTypeStr=Inherit: Inherit via back propagation
  Relational Operator1 : RelationalOperator  Operator=<  OutDataTypeStr=boolean  RndMeth=Simplest
  Switch1 : Switch  Criteria=u2 ~= 0  OutDataTypeStr=Inherit: Inherit via back propagation  RndMeth=Simplest
  Switch2 : Switch  Criteria=u2 ~= 0  OutDataTypeStr=Inherit: Inherit via back propagation  RndMeth=Simplest
  UnitDelay : UnitDelay  InitialCondition=z_cntMaxLim  SampleTime=-1
      settings: AttributesFormatString=Ini=%<X0>
  y : Outport
  wires:
  Switch1/1 -> y/1
  u/1 -> UnitDelay/1
  rst/1 -> Switch1/2
  Constant23/1 -> Switch1/1
  UnitDelay/1 -> Switch2/1, Relational Operator1/1
  Constant1/1 -> Switch2/3, Relational Operator1/2
  Relational Operator1/1 -> Switch2/2
  Switch2/1 -> Switch1/3

== system BLDC_controller_Lib/Debounce_Filter/Default ==
  note: Hold the previous value
  yPrev : Inport
  Action Port : ActionPort
  yDefault : Outport
  wires:
  yPrev/1 -> yDefault/1

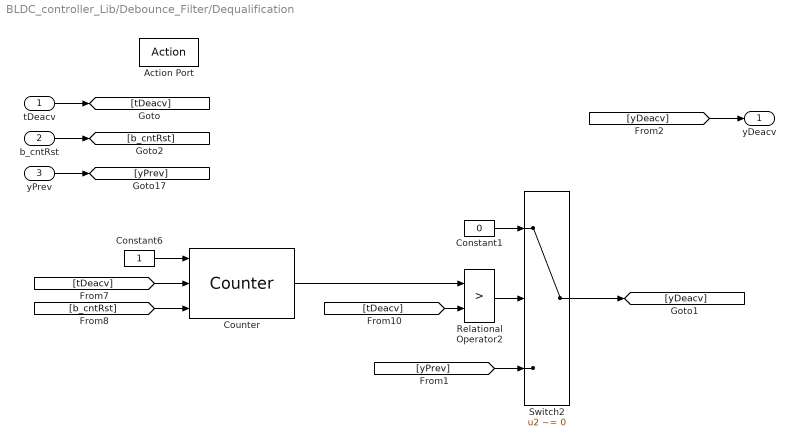
== system BLDC_controller_Lib/Debounce_Filter/Dequalification ==
  tDeacv : Inport
  b_cntRst : Inport  Port=2
  yPrev : Inport  Port=3
  Action Port : ActionPort
  Constant1 : Constant  Value=0  OutDataTypeStr=Inherit: Inherit via back propagation
  Constant6 : Constant  OutDataTypeStr=uint16
  Counter : BLDC_controller_Lib/Counter  z_cntInit=0
  Relational Operator2 : RelationalOperator  Operator=>  OutDataTypeStr=boolean  RndMeth=Simplest
  Switch2 : Switch  Criteria=u2 ~= 0  OutDataTypeStr=Inherit: Inherit via back propagation  RndMeth=Zero
  yDeacv : Outport
  wires:
  Counter/1 -> Relational Operator2/1
  Switch2/1 -> [yDeacv]
  [yPrev] -> Switch2/3
  Constant1/1 -> Switch2/1
  Relational Operator2/1 -> Switch2/2
  [tDeacv] -> Relational Operator2/2
  [b_cntRst] -> Counter/3
  [tDeacv] -> Counter/2
  Constant6/1 -> Counter/1
  yPrev/1 -> [yPrev]
  b_cntRst/1 -> [b_cntRst]
  tDeacv/1 -> [tDeacv]
  [yDeacv] -> yDeacv/1

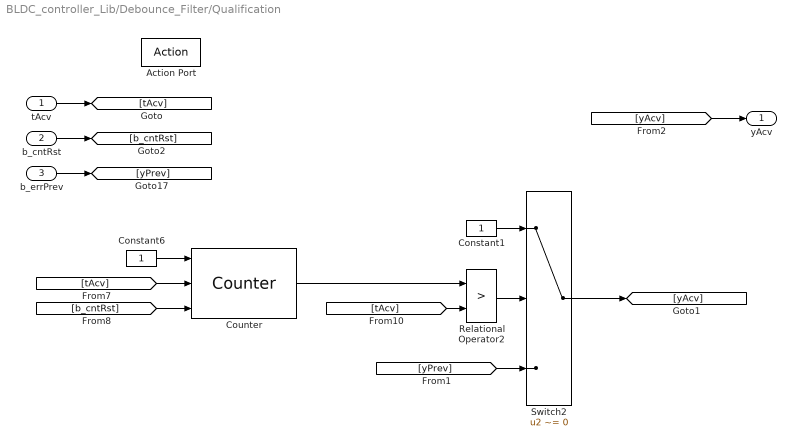
== system BLDC_controller_Lib/Debounce_Filter/Qualification ==
  tAcv : Inport
  b_cntRst : Inport  Port=2
  b_errPrev : Inport  Port=3
  Action Port : ActionPort
  Constant1 : Constant  OutDataTypeStr=Inherit: Inherit via back propagation
  Constant6 : Constant  OutDataTypeStr=uint16
  Counter : BLDC_controller_Lib/Counter  z_cntInit=0
  Relational Operator2 : RelationalOperator  Operator=>  OutDataTypeStr=boolean  RndMeth=Simplest
  Switch2 : Switch  Criteria=u2 ~= 0  OutDataTypeStr=Inherit: Inherit via back propagation  RndMeth=Zero
  yAcv : Outport
  wires:
  [yAcv] -> yAcv/1
  tAcv/1 -> [tAcv]
  b_cntRst/1 -> [b_cntRst]
  b_errPrev/1 -> [yPrev]
  Constant6/1 -> Counter/1
  [tAcv] -> Counter/2
  [b_cntRst] -> Counter/3
  [tAcv] -> Relational Operator2/2
  Relational Operator2/1 -> Switch2/2
  Constant1/1 -> Switch2/1
  [yPrev] -> Switch2/3
  Switch2/1 -> [yAcv]
  Counter/1 -> Relational Operator2/1

== system BLDC_controller_Lib/I_backCalc_fixdt/Integrator ==
  u : Inport
  Data Type Conversion1 : DataTypeConversion  OutDataTypeStr=fixdt(1,16,4)
  Sum1 : Sum  Inputs=|++  RndMeth=Simplest  OutDataTypeStr=Inherit: Same as first input
  UnitDelay : UnitDelay  InitialCondition=yInit  SampleTime=-1
      settings: AttributesFormatString=Ini=%<X0>
  y : Outport
  wires:
  Data Type Conversion1/1 -> y/1
  UnitDelay/1 -> Sum1/2
  Sum1/1 -> UnitDelay/1, Data Type Conversion1/1
  u/1 -> Sum1/1

== system BLDC_controller_Lib/PI_backCalc/Integrator ==
  u : Inport
  Sum1 : Sum  Inputs=|++  RndMeth=Simplest  OutDataTypeStr=Inherit: Same as first input
  UnitDelay : UnitDelay  SampleTime=-1
      settings: AttributesFormatString=Ini=%<X0>
  y : Outport
  wires:
  u/1 -> Sum1/1
  Sum1/1 -> UnitDelay/1, y/1
  UnitDelay/1 -> Sum1/2

== system BLDC_controller_Lib/PI_backCalcTR_fixdt/Integrator ==
  u : Inport
  Sum1 : Sum  Inputs=|++  RndMeth=Simplest  OutDataTypeStr=Inherit: Same as first input
  UnitDelay : UnitDelay  SampleTime=-1
      settings: AttributesFormatString=Ini=%<X0>
  y : Outport
  wires:
  UnitDelay/1 -> Sum1/2
  Sum1/1 -> UnitDelay/1, y/1
  u/1 -> Sum1/1

== system BLDC_controller_Lib/PI_backCalc_fixdt/Integrator ==
  u : Inport
  Data Type Conversion1 : DataTypeConversion  OutDataTypeStr=fixdt(1,16,4)
  Sum1 : Sum  Inputs=|++  RndMeth=Simplest  OutDataTypeStr=Inherit: Same as first input
  UnitDelay : UnitDelay  SampleTime=-1
      settings: AttributesFormatString=Ini=%<X0>
  y : Outport
  wires:
  u/1 -> Sum1/1
  Sum1/1 -> UnitDelay/1, Data Type Conversion1/1
  UnitDelay/1 -> Sum1/2
  Data Type Conversion1/1 -> y/1

== system BLDC_controller_Lib/PI_clamp/Clamping circuit ==
  preIntegrator : Inport  DisableCoverage=on
  preSat : Inport  DisableCoverage=on  Port=2
  satMax : Inport  DisableCoverage=on  Port=3
  satMin : Inport  DisableCoverage=on  Port=4
  AND : Logic  DisableCoverage=on
  DataTypeConv1 : DataTypeConversion  DisableCoverage=on  OutDataTypeStr=int8  RndMeth=Zero  LockScale=on
  DataTypeConv2 : DataTypeConversion  DisableCoverage=on  OutDataTypeStr=int8  RndMeth=Zero  LockScale=on
  Dead Zone Dynamic : simulink/Discontinuities/Dead Zone Dynamic
      settings: SourceProductName=Simulink  SourceProductBaseCode=SL
  Equal : RelationalOperator  DisableCoverage=on  Operator===  RndMeth=Zero  InputSameDT=on
  NotEqual : RelationalOperator  DisableCoverage=on  Operator=~=  RndMeth=Nearest  InputSameDT=on
  SignDeltaU : Signum  DisableCoverage=on
  SignDeltaU1 : Signum  DisableCoverage=on
  a_elecPeriod10 : Constant  Value=0  OutDataTypeStr=Inherit: Inherit via back propagation
  Clamp : Outport  DisableCoverage=on
  wires:
  preIntegrator/1 -> SignDeltaU1/1
  Dead Zone Dynamic/1 -> NotEqual/2, SignDeltaU/1
  SignDeltaU/1 -> DataTypeConv1/1
  DataTypeConv1/1 -> Equal/1
  SignDeltaU1/1 -> DataTypeConv2/1
  DataTypeConv2/1 -> Equal/2
  NotEqual/1 -> AND/1
  Equal/1 -> AND/2
  AND/1 -> Clamp/1
  a_elecPeriod10/1 -> NotEqual/1
  preSat/1 -> Dead Zone Dynamic/2
  satMax/1 -> Dead Zone Dynamic/1
  satMin/1 -> Dead Zone Dynamic/3

== system BLDC_controller_Lib/PI_clamp/Integrator ==
  u : Inport
  Ts : Inport  Port=2
  Divide2 : Product  Inputs=**  OutDataTypeStr=Inherit: Inherit via back propagation  RndMeth=Simplest
  Sum1 : Sum  Inputs=|++  RndMeth=Simplest  OutDataTypeStr=Inherit: Same as first input
  UnitDelay : UnitDelay  SampleTime=-1
      settings: AttributesFormatString=Ini=%<X0>
  y : Outport
  wires:
  UnitDelay/1 -> Sum1/2
  u/1 -> Divide2/1
  Sum1/1 -> UnitDelay/1, y/1
  Divide2/1 -> Sum1/1
  Ts/1 -> Divide2/2

== system BLDC_controller_Lib/PI_clamp_fixdt/Clamping_circuit ==
  preIntegrator : Inport  DisableCoverage=on
  preSat : Inport  DisableCoverage=on  Port=2
  hitSat : Inport  DisableCoverage=on  Port=3
  AND1 : Logic  DisableCoverage=on  OutDataTypeStr=boolean
  DataTypeConv3 : DataTypeConversion  DisableCoverage=on  OutDataTypeStr=int8  RndMeth=Zero  LockScale=on
  DataTypeConv4 : DataTypeConversion  DisableCoverage=on  OutDataTypeStr=int8  RndMeth=Zero  LockScale=on
  Equal1 : RelationalOperator  DisableCoverage=on  Operator===  RndMeth=Zero  InputSameDT=on
  SignDeltaU2 : Signum  DisableCoverage=on
  SignDeltaU3 : Signum  DisableCoverage=on
  Clamp : Outport  DisableCoverage=on
  wires:
  preIntegrator/1 -> SignDeltaU2/1
  preSat/1 -> SignDeltaU3/1
  SignDeltaU2/1 -> DataTypeConv3/1
  SignDeltaU3/1 -> DataTypeConv4/1
  DataTypeConv3/1 -> Equal1/1
  DataTypeConv4/1 -> Equal1/2
  Equal1/1 -> AND1/1
  AND1/1 -> Clamp/1
  hitSat/1 -> AND1/2

== system BLDC_controller_Lib/PI_clamp_fixdt/Integrator ==
  u : Inport
  init : Inport  Port=2
  Data Type Conversion1 : DataTypeConversion  OutDataTypeStr=fixdt(1,16,4)
  Resettable Delay : Delay  DelayLength=1  InitialConditionSource=Input port
      settings: InputPortMap=u0,p4
  Sum1 : Sum  Inputs=|++  RndMeth=Simplest  OutDataTypeStr=Inherit: Same as first input
  y : Outport
  wires:
  u/1 -> Sum1/1
  Sum1/1 -> Resettable Delay/1, Data Type Conversion1/1
  Resettable Delay/1 -> Sum1/2
  Data Type Conversion1/1 -> y/1
  init/1 -> Resettable Delay/2

== system BLDC_controller_Lib/PI_clamp_fixdt_temp/Clamping circuit ==
  preIntegrator : Inport  DisableCoverage=on
  preSat : Inport  DisableCoverage=on  Port=2
  satMax : Inport  DisableCoverage=on  Port=3
  satMin : Inport  DisableCoverage=on  Port=4
  AND : Logic  DisableCoverage=on
  DataTypeConv1 : DataTypeConversion  DisableCoverage=on  OutDataTypeStr=int8  RndMeth=Zero  LockScale=on
  DataTypeConv2 : DataTypeConversion  DisableCoverage=on  OutDataTypeStr=int8  RndMeth=Zero  LockScale=on
  Dead Zone Dynamic : simulink/Discontinuities/Dead Zone Dynamic
      settings: SourceProductName=Simulink  SourceProductBaseCode=SL
  Equal : RelationalOperator  DisableCoverage=on  Operator===  RndMeth=Zero  InputSameDT=on
  NotEqual : RelationalOperator  DisableCoverage=on  Operator=~=  RndMeth=Nearest  InputSameDT=on
  SignDeltaU : Signum  DisableCoverage=on
  SignDeltaU1 : Signum  DisableCoverage=on
  a_elecPeriod10 : Constant  Value=0  OutDataTypeStr=Inherit: Inherit via back propagation
  Clamp : Outport  DisableCoverage=on
  wires:
  satMin/1 -> Dead Zone Dynamic/3
  satMax/1 -> Dead Zone Dynamic/1
  preSat/1 -> Dead Zone Dynamic/2
  a_elecPeriod10/1 -> NotEqual/1
  AND/1 -> Clamp/1
  Equal/1 -> AND/2
  NotEqual/1 -> AND/1
  DataTypeConv2/1 -> Equal/2
  SignDeltaU1/1 -> DataTypeConv2/1
  DataTypeConv1/1 -> Equal/1
  SignDeltaU/1 -> DataTypeConv1/1
  Dead Zone Dynamic/1 -> SignDeltaU/1, NotEqual/2
  preIntegrator/1 -> SignDeltaU1/1

== system BLDC_controller_Lib/PI_clamp_fixdt_temp/Integrator ==
  u : Inport
  Ts : Inport  Port=2
  Divide2 : Product  Inputs=**  OutDataTypeStr=Inherit: Inherit via back propagation  RndMeth=Simplest
  Sum1 : Sum  Inputs=|++  RndMeth=Simplest  OutDataTypeStr=Inherit: Same as first input
  UnitDelay : UnitDelay  SampleTime=-1
      settings: AttributesFormatString=Ini=%<X0>
  y : Outport
  wires:
  UnitDelay/1 -> Sum1/2
  u/1 -> Divide2/1
  Sum1/1 -> UnitDelay/1, y/1
  Divide2/1 -> Sum1/1
  Ts/1 -> Divide2/2

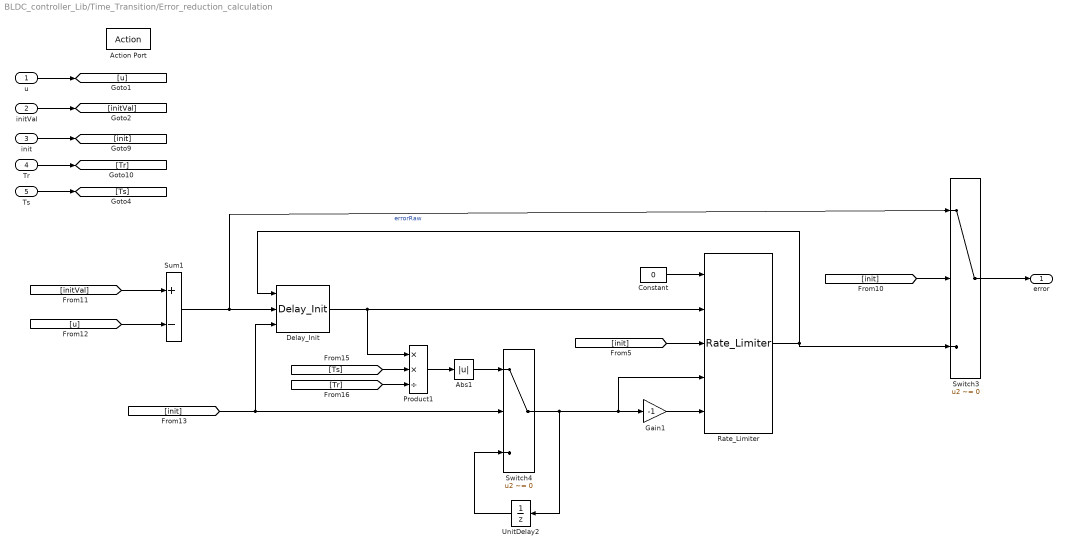
== system BLDC_controller_Lib/Time_Transition/Error_reduction_calculation ==
  u : Inport
  initVal : Inport  Port=2
  init : Inport  Port=3
  Tr : Inport  Port=4
  Ts : Inport  Port=5
  Action Port : ActionPort  InitializeStates=reset
  Abs1 : Abs  RndMeth=Zero  SaturateOnIntegerOverflow=on
  Constant : Constant  Value=0  OutDataTypeStr=Inherit: Inherit via back propagation
  Delay_Init : BLDC_controller_Lib/Delay_Init  initVal=0
      settings: AttributesFormatString=Ini=%<initVal>
  Gain1 : Gain  Gain=-1  RndMeth=Zero  OutDataTypeStr=Inherit: Same as input
  Product1 : Product  Tag=struct('comment',struct('text','','placement',1),'logdata',struct('maxnumvals',inf,'plotchannels',[],'loggingmode',3,'channels',1),'output',struct('variable','','description','','name','$S_$B','width',1,'address','','max',NaN,'min',NaN,'class','default','type','CONTINUOUS','scaling','','lsb',1,'offset',0,'arb',0,'freeze',1,'unit','','autoscalingmode',1,'lowerheadroom',1,'upperheadroom',1,'headroomunit','bit','keepdatatype',1,'checkmin',0,'checkmax',0,'castoutput',0,'show',0),'inputs','**','exceptionhandling',1,'scalingvalid',0,'date',730486)  Inputs=**/  SaturateOnIntegerOverflow=on  RndMeth=Zero
  Rate_Limiter : BLDC_controller_Lib/Rate_Limiter  SystemSampleTime=-1
  Sum1 : Sum  Inputs=+-  RndMeth=Zero  OutDataTypeStr=Inherit: Same as first input
  Switch3 : Switch  Criteria=u2 ~= 0  OutDataTypeStr=Inherit: Inherit via back propagation  RndMeth=Simplest  InputSameDT=on
      settings: AttributesFormatString=Criteria=%<Criteria>
  Switch4 : Switch  Criteria=u2 ~= 0  OutDataTypeStr=Inherit: Inherit via back propagation  RndMeth=Simplest  InputSameDT=on
      settings: AttributesFormatString=Criteria=%<Criteria>
  UnitDelay2 : UnitDelay  SampleTime=-1
      settings: AttributesFormatString=Ini=%<X0>
  error : Outport  OutputWhenDisabled=reset  InitialOutput=0
  wires:
  initVal/1 -> [initVal]
  init/1 -> [init]
  u/1 -> [u]
  Tr/1 -> [Tr]
  Constant/1 -> Rate_Limiter/1
  [init] -> Rate_Limiter/3
  Rate_Limiter/1 -> Delay_Init/1, Switch3/3
  [init] -> Switch3/2
  [initVal] -> Sum1/1
  [u] -> Sum1/2
  Sum1/1 -> Switch3/1, Delay_Init/2  "errorRaw"
  [init] -> Switch4/2, Delay_Init/3
  Delay_Init/1 -> Product1/1, Rate_Limiter/2
  UnitDelay2/1 -> Switch4/3
  Product1/1 -> Abs1/1
  Ts/1 -> [Ts]
  [Ts] -> Product1/2
  [Tr] -> Product1/3
  Switch4/1 -> Rate_Limiter/4, Gain1/1, UnitDelay2/1
  Gain1/1 -> Rate_Limiter/5
  Switch3/1 -> error/1
  Abs1/1 -> Switch4/1
